simulink model "V2X_Core_SRI_coding_rate_symbol"  (R2023b)
settings: Solver=ode23tb  StartTime=0.0  StopTime=50  MaxStep=1e-2  RelTol=1e-3  AbsTol=1e-3
StopFcn:
  | run('saving.m')
values from neighbouring files (symbols this model uses):
  b = 1.6    [a2024_v2x_matlab_6veh.m]
  m = 2000    [a2024_v2x_matlab_6veh.m]
  mEgo = 1500    [a2024_v2x_matlab_6veh.m]
  Mode = 1    [a2024_v2x_matlab_6veh.m]    (also in v2x_matlab.m; v2x_matlabV2.m; v2x_matlab_6veh.m; v2x_matlab_R.m)
  RefSpeed = 90/3.6    (= 25)    [v2x_matlabV2.m]    (also in v2x_matlab_R.m)
  RelDistThreshold = 300    [v2x_matlabV2.m]    (also in v2x_matlab_R.m)
  s = RandStream("dsfmt19937","Seed",15)    [v2x_matlab.m]
  sampleTime = 0.1    [a2024_v2x_matlab_6veh.m]    (also in v2x_matlab.m; v2x_matlabV2.m; v2x_matlab_6veh.m; v2x_matlab_R.m)
  waypoints = [egoWP(:,2) egoWP(:,1), zeroforwp]    [a2024_v2x_matlab_6veh.m]    (also in misc.m = data.data.ActorSpecifications(1,1).Waypoints(:,[1,2]); v2x_matlab.m = data.data.ActorSpecifications(1,1).Waypoints(:,[1,2]); v2x_matlabV2.m = [5 -1.6 0; v2x_matlab_R.m = [5 -1.6 0)
  ZeroActors = struct(     'ActorID',0,     'Position', [1000 1000 1000],      'Velocity', [0 0 0],      'Roll', 0,      'Pitch', 0,      'Yaw', 0,      'AngularVelocity', [0 0 0])    [v2x_matlabV2.m]    (also in v2x_matlab_R.m)
undefined symbols (not defined in the file or in its folder): Battery, Brakes, Control, DiscIntNeverNeededParam, doppler, Drivetrain, ElectricMotor, Env, FB_flag, Init, SNR_value_list, Vehicle, Wheels
libraries: simulink x45, commofdm x29, commdigbbndam3 x15, commchan3 x14, simulink_extras x13, commcnvcod2 x12, commdigbbndpm3 x11, commblkintrlv2 x10, dspmathops x6, sharedtransform x6, autolibutils x6, autolibsharedcoupling x4
(part 4 of 8)

== system V2X_Core_SRI_coding_rate_symbol/DSRC/Subsystem7 ==
  VehicleID : Inport
  Trigger : Inport  Port=2
  Actors : Inport  Port=3
  Ego : Inport  Port=4
  Pilot1 : Inport  Port=5
  1/2 QPSK : Subsystem  Commented=on  TreatAsAtomicUnit=on
  64 QAM : Subsystem  Commented=on  TreatAsAtomicUnit=on
  Add : Sum  Commented=on  Inputs=+-
  Bus Creator : BusCreator  Inputs=2
  Bus Selector : BusSelector  Commented=on  OutputSignals=Actors
  Bus Selector1 : BusSelector  Commented=on  OutputSignals=Position,Velocity
  Constant : Constant  Commented=on  Value=0
  Integer to Bit Converter2 : simulink/Logic and Bit Operations/Integer to Bit Converter  Commented=on  nbits=16  signedInputValues=Signed  bitOrder=MSB first  outDtype=boolean
  MATLAB Function1 : MATLAB Function  Commented=on  TreatAsAtomicUnit=on
  MATLAB Function2 : MATLAB Function  Commented=on  TreatAsAtomicUnit=on
  MATLAB Function3 : MATLAB Function  Commented=on  TreatAsAtomicUnit=on  SystemSampleTime=0.01
  MIMO Fading Channel : commchan3/MIMO Fading Channel  Commented=on  InheritSampleRate=on  SampleRate=1  PathDelays=0  AveragePathGains=0  NormalizePathGains=on  FadingDistribution=Rayleigh  KFactor=3  DirectPathDopplerShift=0  DirectPathInitialPhase=0  MaximumDopplerShift=0.001  DopplerSpectrum=doppler('Jakes')  SpatialCorrelationSpecification=None  SpatialCorrelationMatrix=[1 0 0 0; 0 1 0 0; 0 0 1 0; 0 0 0 1]  NumTransmitAntennas=1  NumReceiveAntennas=1  TransmitCorrelationMatrix=[1 0; 0 1]  ReceiveCorrelationMatrix=[1 0; 0 1]  AntennaSelection=Off  NormalizeChannelOutputs=on  PathGainsOutputPort=off  SimulateUsing=Interpreted execution  FadingTechnique=Filtered Gaussian noise  NumSinusoids=48  InitialTimeSource=Property  InitialTime=0  RandomStream=mt19937ar with seed  Seed=73  Visualization=Off  AntennaPairsToDisplay=[ 1, 1 ]  PathsForDopplerDisplay=1  SamplesToDisplay=25%
  SISO Fading Channel : commchan3/SISO Fading Channel  Commented=on  InheritSampleRate=off  SampleRate=5.9e9  PathDelays=0  AveragePathGains=0  NormalizePathGains=on  FadingDistribution=Rayleigh  KFactor=3  DirectPathDopplerShift=0  DirectPathInitialPhase=0  MaximumDopplerShift=0.001  DopplerSpectrum=doppler('Jakes')  RandomStream=mt19937ar with seed  Seed=73  PathGainsOutputPort=off  ChannelFilterDelayOutputPort=off  SimulateUsing=Interpreted execution  Visualization=Off  PathsForDopplerDisplay=1  SamplesToDisplay=25%
  Scope : Scope  Commented=on
  Scope1 : Scope  Commented=on
  Selector : Selector  Commented=on  InputPortWidth=1  IndexOptions=Index vector (dialog)  Indices=1  OutputSizes=1
  Selector1 : Selector  Commented=on  InputPortWidth=3  IndexOptions=Index vector (dialog)  Indices=1  OutputSizes=1
  Selector2 : Selector  Commented=on  InputPortWidth=3  IndexOptions=Index vector (dialog)  Indices=1  OutputSizes=1
  Variant Sink : VariantSink  Commented=on
  Variant Source : VariantSource  Commented=on
  dB Conversion : dspmathops/dB Conversion  Commented=on  dBtype=dB  intype=Amplitude  R=1  fuzz=off
      settings: LibrarySourceBlock=commutil2/dB Conversion
  SentValues : Outport
  VehicleData : Outport  Port=2
  V1 : Outport  Port=3
  PosX : Outport  Port=4
  VelX : Outport  Port=5
  Actor5 : Outport  Port=6
  wires:
  MATLAB Function1/1(Actor) -> MATLAB Function3/1(input), Integer to Bit Converter2/1
  Ego/1 -> MATLAB Function1/3(EgoData)
  Actors/1 -> Bus Selector/1, MATLAB Function1/1(busActors3Test1)
  VehicleID/1 -> MATLAB Function1/2(VehicleID)
  MATLAB Function1/2(VehicleData) -> VehicleData/1
  MATLAB Function1/3(counter_out) -> V1/1
  Trigger/1 -> MATLAB Function1/Trigger
  MATLAB Function1/5(Pr) -> Bus Creator/2, Scope1/1  "ActorRxPower"
  MATLAB Function1/4(SNR) -> Add/1
  Add/1 -> MATLAB Function2/2(SNR), Scope/1
  Selector1/1 -> PosX/1
  Bus Selector/1 -> Selector/1  "<Actors>"
  Selector/1 -> Bus Selector1/1
  Bus Selector1/1 -> Selector1/1  "<Position>"
  Bus Selector1/2 -> Selector2/1  "<Velocity>"
  Selector2/1 -> VelX/1
  Variant Sink/2 -> 1/2 QPSK/1(Bits)
  Pilot1/1 -> 64 QAM/2(Pilot), 1/2 QPSK/2(Pilot)
  Integer to Bit Converter2/1 -> Variant Sink/1
  Variant Source/1 -> MATLAB Function2/1(modulated)
  1/2 QPSK/1(Modulated) -> Variant Source/2
  64 QAM/1(Modulated) -> Variant Source/1
  Variant Sink/1 -> 64 QAM/1(Bits)
  Constant/1 -> Add/2
  MATLAB Function2/1(signal) -> Bus Creator/1  "ActorData"
  Bus Creator/1 -> Actor5/1
  MATLAB Function3/1(Actors) -> SentValues/1

== system V2X_Core_SRI_coding_rate_symbol/DSRC/Subsystem8 ==
  VehicleID : Inport
  Trigger : Inport  Port=2
  Actors : Inport  Port=3
  Ego : Inport  Port=4
  Pilot1 : Inport  Port=5
  1/2 QPSK : Subsystem  Commented=on  TreatAsAtomicUnit=on
  64 QAM : Subsystem  Commented=on  TreatAsAtomicUnit=on
  Add : Sum  Commented=on  Inputs=+-
  Bus Creator : BusCreator  Inputs=2
  Bus Selector : BusSelector  Commented=on  OutputSignals=Actors
  Bus Selector1 : BusSelector  Commented=on  OutputSignals=Position,Velocity
  Constant : Constant  Commented=on  Value=0
  Integer to Bit Converter2 : simulink/Logic and Bit Operations/Integer to Bit Converter  Commented=on  nbits=16  signedInputValues=Signed  bitOrder=MSB first  outDtype=boolean
  MATLAB Function1 : MATLAB Function  Commented=on  TreatAsAtomicUnit=on
  MATLAB Function2 : MATLAB Function  Commented=on  TreatAsAtomicUnit=on
  MATLAB Function3 : MATLAB Function  Commented=on  TreatAsAtomicUnit=on  SystemSampleTime=0.01
  MIMO Fading Channel : commchan3/MIMO Fading Channel  Commented=on  InheritSampleRate=on  SampleRate=1  PathDelays=0  AveragePathGains=0  NormalizePathGains=on  FadingDistribution=Rayleigh  KFactor=3  DirectPathDopplerShift=0  DirectPathInitialPhase=0  MaximumDopplerShift=0.001  DopplerSpectrum=doppler('Jakes')  SpatialCorrelationSpecification=None  SpatialCorrelationMatrix=[1 0 0 0; 0 1 0 0; 0 0 1 0; 0 0 0 1]  NumTransmitAntennas=1  NumReceiveAntennas=1  TransmitCorrelationMatrix=[1 0; 0 1]  ReceiveCorrelationMatrix=[1 0; 0 1]  AntennaSelection=Off  NormalizeChannelOutputs=on  PathGainsOutputPort=off  SimulateUsing=Interpreted execution  FadingTechnique=Filtered Gaussian noise  NumSinusoids=48  InitialTimeSource=Property  InitialTime=0  RandomStream=mt19937ar with seed  Seed=73  Visualization=Off  AntennaPairsToDisplay=[ 1, 1 ]  PathsForDopplerDisplay=1  SamplesToDisplay=25%
  SISO Fading Channel : commchan3/SISO Fading Channel  Commented=on  InheritSampleRate=off  SampleRate=5.9e9  PathDelays=0  AveragePathGains=0  NormalizePathGains=on  FadingDistribution=Rayleigh  KFactor=3  DirectPathDopplerShift=0  DirectPathInitialPhase=0  MaximumDopplerShift=0.001  DopplerSpectrum=doppler('Jakes')  RandomStream=mt19937ar with seed  Seed=73  PathGainsOutputPort=off  ChannelFilterDelayOutputPort=off  SimulateUsing=Interpreted execution  Visualization=Off  PathsForDopplerDisplay=1  SamplesToDisplay=25%
  Scope : Scope  Commented=on
  Scope1 : Scope  Commented=on
  Selector : Selector  Commented=on  InputPortWidth=1  IndexOptions=Index vector (dialog)  Indices=1  OutputSizes=1
  Selector1 : Selector  Commented=on  InputPortWidth=3  IndexOptions=Index vector (dialog)  Indices=1  OutputSizes=1
  Selector2 : Selector  Commented=on  InputPortWidth=3  IndexOptions=Index vector (dialog)  Indices=1  OutputSizes=1
  Variant Sink : VariantSink  Commented=on
  Variant Source : VariantSource  Commented=on
  dB Conversion : dspmathops/dB Conversion  Commented=on  dBtype=dB  intype=Amplitude  R=1  fuzz=off
      settings: LibrarySourceBlock=commutil2/dB Conversion
  SentValues : Outport
  VehicleData : Outport  Port=2
  V1 : Outport  Port=3
  PosX : Outport  Port=4
  VelX : Outport  Port=5
  Actor6 : Outport  Port=6
  wires:
  MATLAB Function3/1(Actors) -> SentValues/1
  Bus Creator/1 -> Actor6/1
  MATLAB Function2/1(signal) -> Bus Creator/1  "ActorData"
  Constant/1 -> Add/2
  Variant Sink/1 -> 64 QAM/1(Bits)
  64 QAM/1(Modulated) -> Variant Source/1
  1/2 QPSK/1(Modulated) -> Variant Source/2
  Variant Source/1 -> MATLAB Function2/1(modulated)
  Integer to Bit Converter2/1 -> Variant Sink/1
  Pilot1/1 -> 1/2 QPSK/2(Pilot), 64 QAM/2(Pilot)
  Variant Sink/2 -> 1/2 QPSK/1(Bits)
  Selector2/1 -> VelX/1
  Bus Selector1/2 -> Selector2/1  "<Velocity>"
  Bus Selector1/1 -> Selector1/1  "<Position>"
  Selector/1 -> Bus Selector1/1
  Bus Selector/1 -> Selector/1  "<Actors>"
  Selector1/1 -> PosX/1
  Add/1 -> Scope/1, MATLAB Function2/2(SNR)
  MATLAB Function1/4(SNR) -> Add/1
  MATLAB Function1/5(Pr) -> Scope1/1, Bus Creator/2  "ActorRxPower"
  Trigger/1 -> MATLAB Function1/Trigger
  MATLAB Function1/3(counter_out) -> V1/1
  MATLAB Function1/2(VehicleData) -> VehicleData/1
  VehicleID/1 -> MATLAB Function1/2(VehicleID)
  Actors/1 -> MATLAB Function1/1(busActors3Test1), Bus Selector/1
  Ego/1 -> MATLAB Function1/3(EgoData)
  MATLAB Function1/1(Actor) -> Integer to Bit Converter2/1, MATLAB Function3/1(input)

== system V2X_Core_SRI_coding_rate_symbol/DelayMessage1/Subsystem ==
  Queue : Inport
  Trigger : TriggerPort  VariantControl=(inherit)  PortDimensions=1
  Receive : Receive  InputPortMessageModes=m  UseInternalQueue=off  QueueOverwriting=on  QueueLength=1  QueueType=LIFO
  Out : Outport
  wires:
  Queue/1 -> Receive/1
  Receive/1 -> Out/1

== system V2X_Core_SRI_coding_rate_symbol/VehicleDynamic/AccelerationToTrq ==
  IntendedLongAcc[m/s**2] : Inport
  LongVehSpd[m/s] : Inport  Port=2
  UnloadedTireRadius[m] : Inport  Port=3
  OverallMass[kg] : Inport  Port=4
  EngInrt[kg*m**2] : Inport  Port=5
  WheelRotAxisInrt[kg*m**2] : Inport  Port=6
  TireMaxRollResistanceTrq[Nm] : Inport  Port=7
  AeroFrc(VehSys)[N] : Inport  Port=8
  TorqueRatio[-] : Inport  Port=9
  ZeroAccPedalTrq[Nm] : Inport  Port=10
  FullAccPedalTrq[Nm] : Inport  Port=11
  StandstillSwitch[0;1] : Inport  Port=12
  MaxMainBrakePress[Pa] : Inport  Port=13
  BrakeTrqPressRatio[m**3] : Inport  Port=14
  CalculateIntendedTorque : Subsystem
  CalculateMainBrakePressure : Subsystem
  Scope : Scope
  TorqueSplitter : Subsystem
  IntendedDriveTrq[Nm] : Outport
  IntendedMainBrakePress[Pa] : Outport  Port=2
  IntendedTrq[Nm] : Outport  Port=3
  wires:
  EngInrt[kg*m**2]/1 -> CalculateIntendedTorque/4(EngInrt[kg*m**2])
  TorqueSplitter/2(IntendedBrakeTrq[Nm]) -> CalculateMainBrakePressure/1(IntendedBrakeTrq[Nm])
  OverallMass[kg]/1 -> CalculateIntendedTorque/3(OverallMass[kg])
  FullAccPedalTrq[Nm]/1 -> TorqueSplitter/4(FullAccPedalTrq[Nm])
  TorqueRatio[-]/1 -> TorqueSplitter/3(TorqueRatio[-]), CalculateIntendedTorque/8(TorqueRatio[-])
  StandstillSwitch[0;1]/1 -> CalculateMainBrakePressure/2(StandstillSwitch[0;1])
  TireMaxRollResistanceTrq[Nm]/1 -> CalculateIntendedTorque/6(TireMaxRollResistanceTrq[Nm])
  IntendedLongAcc[m/s**2]/1 -> CalculateIntendedTorque/1(IntendedLongAcc[m/s**2])
  ZeroAccPedalTrq[Nm]/1 -> TorqueSplitter/2(ZeroAccPedalTrq[Nm]), CalculateIntendedTorque/9(MinEngTrq[Nm])
  UnloadedTireRadius[m]/1 -> CalculateIntendedTorque/2(UnloadedTireRadius[m])
  TorqueSplitter/1(IntendedDriveTrq[Nm]) -> IntendedDriveTrq[Nm]/1
  LongVehSpd[m/s]/1 -> CalculateMainBrakePressure/3(LongVehSpd[m/s])
  BrakeTrqPressRatio[m**3]/1 -> CalculateMainBrakePressure/5(BrakeTrqPressRatio[m**3])
  WheelRotAxisInrt[kg*m**2]/1 -> CalculateIntendedTorque/5(WheelRotAxisInrt[kg*m**2])
  MaxMainBrakePress[Pa]/1 -> CalculateMainBrakePressure/4(MaxMainBrakePress[Pa])
  AeroFrc(VehSys)[N]/1 -> CalculateIntendedTorque/7(AeroFrc(VehSys)[N])
  CalculateMainBrakePressure/1(IntendedMainBrakePress[Pa]) -> Scope/1, IntendedMainBrakePress[Pa]/1
  CalculateIntendedTorque/1(IntendedTrq[Nm]) -> IntendedTrq[Nm]/1, TorqueSplitter/1("IntendedTrq[Nm] ")

== system V2X_Core_SRI_coding_rate_symbol/VehicleDynamic/DrivetrainControlUnit ==
  note: Copyright 2015-2022 The MathWorks, Inc.
  AccelPdl : Inport  OutDataTypeStr=double  PortDimensions=1
  BcuBrkPrsCmd : Inport  Port=2  OutDataTypeStr=double  PortDimensions=4
  VehSpdFdbk : Inport  Port=3  OutDataTypeStr=double  PortDimensions=1
  EMSpd : Inport  Port=4  OutDataTypeStr=double  PortDimensions=1
  BMSSOC : Inport  Port=5
  BattPackVolt : Inport  Port=6
  BMSDischrgCurrLmt : Inport  Port=7
  BMSChrgCurrLmt : Inport  Port=8
  IntendedDriveTrq[Nm] : Inport  Port=9
  Accel Pedal to Traction Wheel Torque Request : Subsystem  InitFcn=[~]=autosharedicon('autolibinternalvvblock',gcb,0,'6');
  Brake Pedal to Total Braking Pressure Request : Subsystem
  Constant : Constant  Value=0
  Motor Torque Arbitration and Power Management : Subsystem
  Power Limit Calculations : Subsystem
  Series Regen Braking : Subsystem
  Subsystem2 : Subsystem
  Terminator : Terminator
  EMTrqCmd : Outport  OutDataTypeStr=double  PortDimensions=1  VectorParamsAs1DForOutWhenUnconnected=off
  DcuBrkPrsCmd : Outport  Port=2  OutDataTypeStr=double  PortDimensions=4  VectorParamsAs1DForOutWhenUnconnected=off
  wires:
  BMSSOC/1 -> Subsystem2/1(SOC)
  [EMSpd] -> Motor Torque Arbitration and Power Management/5(EMSpd)
  BMSDischrgCurrLmt/1 -> Power Limit Calculations/2(BMSDischrgCurrLmt)
  Series Regen Braking/1(" EMTrqCmdRegen") -> Motor Torque Arbitration and Power Management/7(EMTrqCmdRegen)  "EMTrqCmdRegen"
  Brake Pedal to Total Braking Pressure Request/1(BrkPrsReq) -> Series Regen Braking/4("BrkPrsReq ")
  AccelPdl/1 -> [AccelPdl], Accel Pedal to Traction Wheel Torque Request/1(AccelPdl)
  Constant/1 -> Brake Pedal to Total Braking Pressure Request/2(Park)
  BMSChrgCurrLmt/1 -> Power Limit Calculations/3(BMSChrgCurrLmt)
  BcuBrkPrsCmd/1 -> Brake Pedal to Total Braking Pressure Request/1(BcuBrkPrsCmd)  "DecelPdl"
  BattPackVolt/1 -> Power Limit Calculations/1(PackVolt)
  VehSpdFdbk/1 -> Series Regen Braking/2(VehSpd)  "VehSpd"
  EMSpd/1 -> Series Regen Braking/3("EMSpd "), [EMSpd]  "EMSpd"
  [EMSpd] -> Accel Pedal to Traction Wheel Torque Request/2(EMSpd)
  Power Limit Calculations/2(BattPwrChrgLmt) -> Motor Torque Arbitration and Power Management/4("BattPwrChrgLmt ")  "BattPwrChrgLmt"
  Power Limit Calculations/1(BattPwrDischrgLmt) -> Motor Torque Arbitration and Power Management/3(BattPwrDisChrgLmt)  "BattPwrDischrgLmt"
  [AccelPdl] -> Motor Torque Arbitration and Power Management/2(AccelPdl)
  Motor Torque Arbitration and Power Management/1(EMTrqCmdFinal) -> EMTrqCmd/1  "EMTrqCmd"
  Subsystem2/1(BattSOC) -> Series Regen Braking/1(BattSoc), Motor Torque Arbitration and Power Management/6(SOC)  "SOC"
  IntendedDriveTrq[Nm]/1 -> Motor Torque Arbitration and Power Management/1(EMTrqCmdTrac)
  Accel Pedal to Traction Wheel Torque Request/1(TrqCmd) -> Terminator/1
  Series Regen Braking/2(" BrkCmd") -> DcuBrkPrsCmd/1  "BrkCmd"

== system V2X_Core_SRI_coding_rate_symbol/VehicleDynamic/Enabled Subsystem ==
  In1 : Inport
  Enable : EnablePort
  Out1 : Outport
  wires:
  In1/1 -> Out1/1

== system V2X_Core_SRI_coding_rate_symbol/VehicleDynamic/FiveSteteABS-TCS ==
  note: Copyright 2022 The MathWorks, Inc.
  AccelFdbk : Inport  OutDataTypeStr=double  PortDimensions=1
  DecelFdbk : Inport  Port=2  OutDataTypeStr=double  PortDimensions=1
  Acc : Inport  Port=3  OutDataTypeStr=double
  Omega : Inport  Port=4  OutDataTypeStr=double  PortDimensions=4
  BrkPrs : Inport  Port=5  OutDataTypeStr=double  PortDimensions=4
  ABSCtrlForEach : Subsystem  mask(Five-State ABS Control){Re=Wheels.EffectiveRadius, KappaOpt=-0.12, WhlAccelOpt=[-9.8,-9.8,-20,-20], v1=0, v5=0.55, v4=1, a2=-1.5, b=-1.5, A=4.5, a1=3.6, aMode=2}
      mask prompts: Re "Wheel effective radius, Re [m]:"; KappaOpt "Desired wheel slip ratio, KappaOpt [-]:"; WhlAccelOpt "Desired wheel acceleration, WhlAccelOpt [m/s^2]:"; v1 "Braking realease command, v1 [-]:"; v5 "Braking hold command, v5 [-]:"; v4 "Braking add command, v4 [-]:"; a2 "Threshold of State 1, a2 [m/s^2]:"; b "Threshold of State 2, b [m/s^2]:"; A "Threshold of State 3 and 4, A [m/s^2]:"; a1 "Threshold of State 5, a1 [m/s^2]:"
      mask help: This block determines brake pressure varying rate for each wheel once the ABS controller is activated. During ABS control, only wheel speed is directly regulated.
      mask init:
      | [~]=vehdynicon('vehdynblk',gcb);
      mask DialogControl vehParamGroup Prompt: Vehicle Parameter
      mask DialogControl ParameterGroupVar Prompt: Desired Control Parameters
      mask DialogControl Container3 Prompt: Braking Pressure Rates
      mask DialogControl Container4 Prompt: Wheel Acceleration Thresholds
  Data Type Conversion : DataTypeConversion  OutDataTypeStr=boolean  SaturateOnIntegerOverflow=off  RndMeth=Floor
  Logical Operator : Logic  Operator=OR  AllPortsSameDT=off  OutDataTypeStr=boolean
  Sum : Sum  Inputs=|++
  Switch : Switch  Criteria=u2 > Threshold  SaturateOnIntegerOverflow=off  InputSameDT=off
  TCSCtrlForEach : Subsystem  mask(Five-State TCS Control){Re=Wheels.EffectiveRadius, KappaOpt=0.12, WhlAccelOpt=[11, 11, 11, 11], v1=1.5, v5=-0.5, v4=-1.2, a2=-6, b=-10, A=-11, a1=-9, aMode=2}
      mask prompts: Re "Wheel effective radius, Re [m]:"; KappaOpt "Desired wheel slip ratio, KappaOpt [-]:"; WhlAccelOpt "Desired wheel acceleration, WhlAccelOpt [m/s^2]:"; v1 "Braking pressure rising rate, v1 [-]:"; v5 "Secondary braking pressure declining rate, v5 [-]:"; v4 "Braking pressure declining rate, v4 [-]:"; a2 "Threshold of State 1, a2 [m/s^2]:"; b "Threshold of State 2, b [m/s^2]:"; A "Threshold of State 3 and 4, A [m/s^2]:"; a1 "Threshold of State 5, a1 [m/s^2]:"
      mask help: This block determines brake pressure varying rate for each wheel once the TCS controller is activated. During TCS control, only wheel speed is directly regulated.
      mask init:
      | [~]=vehdynicon('vehdynblk',gcb);
      mask DialogControl vehParamGroup Prompt: Vehicle Parameter
      mask DialogControl ParameterGroupVar Prompt: Desired Control Parameters
      mask DialogControl Container3 Prompt: Braking Pressure Rates
      mask DialogControl Container4 Prompt: Wheel Acceleration Thresholds
  Wheel Accel and Slip Estimator1 : Subsystem
  BrkPrsCmd : Outport  OutDataTypeStr=double  PortDimensions=4
  ABSFlag : Outport  Port=2  OutDataTypeStr=boolean  PortDimensions=4
  TCSFlag : Outport  Port=3  OutDataTypeStr=double  PortDimensions=4
  wires:
  Sum/1 -> Switch/1
  Wheel Accel and Slip Estimator1/2(<Kappa>) -> TCSCtrlForEach/2(WhlSlip), ABSCtrlForEach/3(WhlSlip)
  Wheel Accel and Slip Estimator1/1(<WhlAccel>) -> TCSCtrlForEach/1(WhlAccel), ABSCtrlForEach/2(WhlAccel)
  AccelFdbk/1 -> TCSCtrlForEach/3(AccelFdbk)
  Acc/1 -> Wheel Accel and Slip Estimator1/2(Accel)
  BrkPrs/1 -> TCSCtrlForEach/4(PbFdbk)
  TCSCtrlForEach/2(BrkFlag) -> TCSFlag/1, Logical Operator/2
  ABSCtrlForEach/1(BrkCtrl) -> Sum/1
  ABSCtrlForEach/2(BrkFlag) -> Data Type Conversion/1, Logical Operator/1
  Switch/1 -> BrkPrsCmd/1
  Data Type Conversion/1 -> ABSFlag/1
  Logical Operator/1 -> Switch/2
  Omega/1 -> Wheel Accel and Slip Estimator1/1(Omega)
  TCSCtrlForEach/1(BrkCtrl) -> Sum/2
  Wheel Accel and Slip Estimator1/3(<xdot>) -> ABSCtrlForEach/4(VehSpd)
  DecelFdbk/1 -> Switch/3, ABSCtrlForEach/1(Pref)

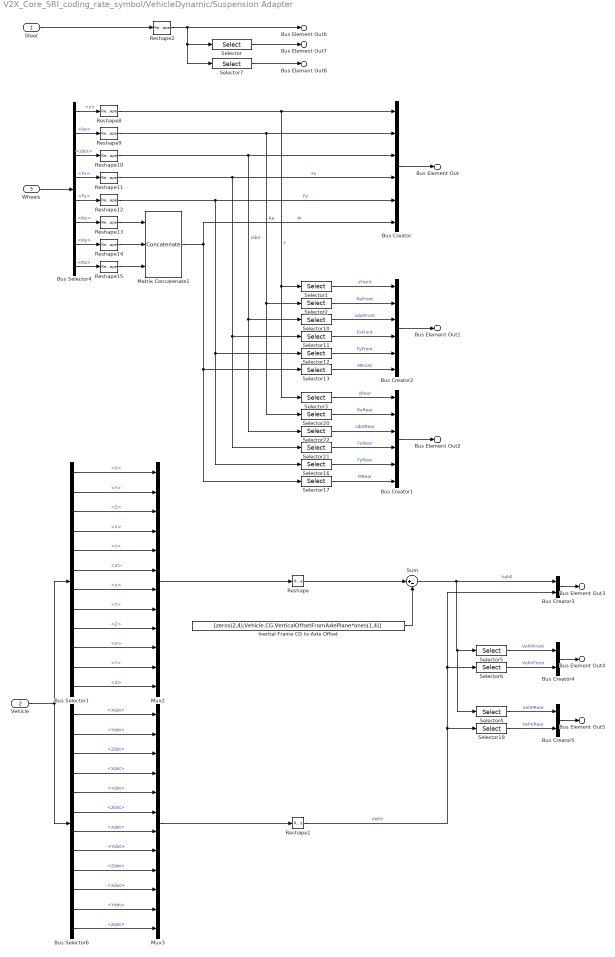
== system V2X_Core_SRI_coding_rate_symbol/VehicleDynamic/Suspension Adapter ==
  Steer : Inport
  Vehicle : Inport  Port=2
  Wheels : Inport  Port=3
  Bus Creator : BusCreator  Inputs=6
  Bus Creator1 : BusCreator  Inputs=6
  Bus Creator2 : BusCreator  Inputs=6
  Bus Creator3 : BusCreator  Inputs=2
  Bus Creator4 : BusCreator  Inputs=2
  Bus Creator5 : BusCreator  Inputs=2
  Bus Selector1 : BusSelector  OutputSignals=InertFrm.FrntAxl.Lft.Disp.X,InertFrm.FrntAxl.Lft.Disp.Y,InertFrm.FrntAxl.Lft.Disp.Z,InertFrm.FrntAxl.Rght.Disp.X,InertFrm.FrntAxl.Rght.Disp.Y,InertFrm.FrntAxl.Rght.Disp.Z,InertFrm.RearAxl.Lft.Disp.X,InertFrm.RearAxl.Lft.Disp.Y,InertFrm.RearAxl.Lft.Disp.Z,InertFrm.RearAxl.Rght.Disp.X,InertFrm.RearAxl.Rght.Disp.Y,InertFrm.RearAxl.Rght.Disp.Z
  Bus Selector4 : BusSelector  OutputSignals=SuspFrame.z,SuspFrame.Re,SuspFrame.zdot,SuspFrame.Fx,SuspFrame.Fy,SuspFrame.Mx,SuspFrame.My,SuspFrame.Mz
  Bus Selector6 : BusSelector  OutputSignals=InertFrm.FrntAxl.Lft.Vel.Xdot,InertFrm.FrntAxl.Lft.Vel.Ydot,InertFrm.FrntAxl.Lft.Vel.Zdot,InertFrm.FrntAxl.Rght.Vel.Xdot,InertFrm.FrntAxl.Rght.Vel.Ydot,InertFrm.FrntAxl.Rght.Vel.Zdot,InertFrm.RearAxl.Lft.Vel.Xdot,InertFrm.RearAxl.Lft.Vel.Ydot,InertFrm.RearAxl.Lft.Vel.Zdot,InertFrm.RearAxl.Rght.Vel.Xdot,InertFrm.RearAxl.Rght.Vel.Ydot,InertFrm.RearAxl.Rght.Vel.Zdot
  Inertial Frame CG to Axle Offset : Constant  Value=[zeros(2,4);Vehicle.CG.VerticalOffsetFromAxlePlane*ones(1,4)]
  Matrix Concatenate1 : Concatenate  NumInputs=3  Mode=Multidimensional array
  Mux2 : Mux  Inputs=12
  Mux3 : Mux  Inputs=12
  Reshape : Reshape  OutputDimensionality=Customize  OutputDimensions=[3,4]
  Reshape1 : Reshape  OutputDimensionality=Customize  OutputDimensions=[3,4]
  Reshape{2,8..15} (9 alike) : Reshape  OutputDimensionality=Row vector (2-D)
  Selector{,1..2,10..12} (6 alike) : Selector  IndexOptions=Index vector (dialog)  Indices=[1 2]  OutputSizes=1
  Selector13 : Selector  NumberOfDimensions=2  IndexOptions=Select all,Index vector (dialog)  Indices=[1 2],[1 2]  OutputSizes=1,1
  Selector{3,7,16,20..22} (6 alike) : Selector  IndexOptions=Index vector (dialog)  Indices=[3 4]  OutputSizes=1
  Selector17 : Selector  NumberOfDimensions=2  IndexOptions=Select all,Index vector (dialog)  Indices=[1 2],[3 4]  OutputSizes=1,1
  Selector18 : Selector  NumberOfDimensions=2  IndexOptions=Select all,Index vector (dialog)  Indices=[1 2],[3 4]  OutputSizes=1,1
  Selector4 : Selector  NumberOfDimensions=2  IndexOptions=Select all,Index vector (dialog)  Indices=[1 2],[3 4]  OutputSizes=1,1
  Selector5 : Selector  NumberOfDimensions=2  IndexOptions=Select all,Index vector (dialog)  Indices=[1 2],[1 2]  OutputSizes=1,1
  Selector6 : Selector  NumberOfDimensions=2  IndexOptions=Select all,Index vector (dialog)  Indices=[1 2],[1 2]  OutputSizes=1,1
  Sum : Sum  Inputs=|+-
  Bus Element Out : Outport  PortName=WheelsSusp  Element=All
  Bus Element Out1 : Outport  PortName=WheelsSusp  Element=Front
  Bus Element Out2 : Outport  PortName=WheelsSusp  Element=Rear
  Bus Element Out3 : Outport  Port=2  PortName=VehSusp  Element=All
  Bus Element Out4 : Outport  Port=2  PortName=VehSusp  Element=Front
  Bus Element Out5 : Outport  Port=2  PortName=VehSusp  Element=Rear
  Bus Element Out6 : Outport  Port=3  PortName=SteeringAngles  Element=StrgAngAll
  Bus Element Out7 : Outport  Port=3  PortName=SteeringAngles  Element=StrgAngFront
  Bus Element Out8 : Outport  Port=3  PortName=SteeringAngles  Element=StrgAngRear
  wires:
  Reshape9/1 -> Selector2/1, Selector20/1, Bus Creator/2  "Re"
  Selector2/1 -> Bus Creator2/2  "ReFront"
  Selector13/1 -> Bus Creator2/6  "MFront"
  Selector11/1 -> Bus Creator2/4  "FxFront"
  Reshape12/1 -> Bus Creator/5, Selector12/1, Selector16/1  "Fy"
  Selector1/1 -> Bus Creator2/1  "zFront"
  Bus Creator/1 -> Bus Element Out/1
  Reshape11/1 -> Bus Creator/4, Selector11/1, Selector21/1  "Fx"
  Bus Creator1/1 -> Bus Element Out2/1
  Selector3/1 -> Bus Creator1/1  "zRear"
  Wheels/1 -> Bus Selector4/1
  Selector12/1 -> Bus Creator2/5  "FyFront"
  Matrix Concatenate1/1 -> Bus Creator/6, Selector13/1, Selector17/1  "M"
  Bus Selector4/5 -> Reshape12/1  "<Fy>"
  Bus Selector4/2 -> Reshape9/1  "<Re>"
  Reshape13/1 -> Matrix Concatenate1/1
  Reshape14/1 -> Matrix Concatenate1/2
  Bus Selector4/1 -> Reshape8/1  "<z>"
  Bus Creator2/1 -> Bus Element Out1/1
  Selector17/1 -> Bus Creator1/6  "MRear"
  Reshape15/1 -> Matrix Concatenate1/3
  Bus Selector4/7 -> Reshape14/1  "<My>"
  Bus Selector4/8 -> Reshape15/1  "<Mz>"
  Bus Selector4/4 -> Reshape11/1  "<Fx>"
  Bus Selector4/3 -> Reshape10/1  "<zdot>"
  Selector10/1 -> Bus Creator2/3  "zdotFront"
  Selector22/1 -> Bus Creator1/3  "zdotRear"
  Reshape10/1 -> Bus Creator/3, Selector10/1, Selector22/1  "zdot"
  Reshape8/1 -> Bus Creator/1, Selector1/1, Selector3/1  "z"
  Selector16/1 -> Bus Creator1/5  "FyRear"
  Selector21/1 -> Bus Creator1/4  "FxRear"
  Bus Selector4/6 -> Reshape13/1  "<Mx>"
  Selector20/1 -> Bus Creator1/2  "ReRear"
  Selector4/1 -> Bus Creator5/1  "VehPRear"
  Bus Creator4/1 -> Bus Element Out4/1
  Bus Selector6/1 -> Mux3/1  "<Xdot>"
  Bus Selector6/9 -> Mux3/9  "<Zdot>"
  Bus Selector1/10 -> Mux2/10  "<X>"
  Bus Selector1/8 -> Mux2/8  "<Y>"
  Reshape1/1 -> Bus Creator3/2, Selector6/1, Selector18/1  "VehV"
  Reshape/1 -> Sum/1
  Mux3/1 -> Reshape1/1
  Bus Selector1/5 -> Mux2/5  "<Y>"
  Bus Selector6/2 -> Mux3/2  "<Ydot>"
  Bus Selector1/2 -> Mux2/2  "<Y>"
  Bus Selector1/4 -> Mux2/4  "<X>"
  Bus Creator5/1 -> Bus Element Out5/1
  Bus Selector1/3 -> Mux2/3  "<Z>"
  Bus Selector1/9 -> Mux2/9  "<Z>"
  Bus Selector1/11 -> Mux2/11  "<Y>"
  Bus Selector6/11 -> Mux3/11  "<Ydot>"
  Bus Selector1/6 -> Mux2/6  "<Z>"
  Bus Selector6/8 -> Mux3/8  "<Ydot>"
  Inertial Frame CG to Axle Offset/1 -> Sum/2
  Bus Selector6/5 -> Mux3/5  "<Ydot>"
  Vehicle/1 -> Bus Selector6/1, Bus Selector1/1
  Bus Selector6/6 -> Mux3/6  "<Zdot>"
  Bus Selector6/10 -> Mux3/10  "<Xdot>"
  Selector18/1 -> Bus Creator5/2  "VehVRear"
  Selector6/1 -> Bus Creator4/2  "VehVFront"
  Bus Selector1/1 -> Mux2/1  "<X>"
  Bus Selector1/12 -> Mux2/12  "<Z>"
  Bus Creator3/1 -> Bus Element Out3/1
  Bus Selector1/7 -> Mux2/7  "<X>"
  Bus Selector6/4 -> Mux3/4  "<Xdot>"
  Selector5/1 -> Bus Creator4/1  "VehPFront"
  Bus Selector6/12 -> Mux3/12  "<Zdot>"
  Bus Selector6/3 -> Mux3/3  "<Zdot>"
  Bus Selector6/7 -> Mux3/7  "<Xdot>"
  Mux2/1 -> Reshape/1
  Sum/1 -> Selector4/1, Selector5/1, Bus Creator3/1  "VehP"
  Steer/1 -> Reshape2/1
  Reshape2/1 -> Selector7/1, Selector/1, Bus Element Out6/1
  Selector7/1 -> Bus Element Out8/1
  Selector/1 -> Bus Element Out7/1

== system V2X_Core_SRI_coding_rate_symbol/VehicleDynamic/Suspension Bus Creator ==
  Vehicle : Inport
  SuspensionInfo : Inport  Port=2
  Wheels : Inport  Port=3
  Add : Sum
  Bus Creator1 : BusCreator  Inputs=6
  Bus Creator2 : BusCreator  Inputs=2
  Bus Creator3 : BusCreator  Inputs=2
  Bus Selector1 : BusSelector  OutputSignals=BdyFrm.Cg.AngVel.r
  Bus Selector2 : BusSelector  OutputSignals=SuspFrame.z
  Bus Selector5 : BusSelector  OutputSignals=Front.VehF,Rear.VehF,Front.VehM,Rear.VehM,Front.WhlF,Rear.WhlF,Front.WhlAng,Rear.WhlAng
  Bus Selector6 : BusSelector  OutputSignals=BdyFrm.FrntAxl.Lft.Vel.xdot,BdyFrm.FrntAxl.Rght.Vel.xdot,BdyFrm.RearAxl.Lft.Vel.xdot,BdyFrm.RearAxl.Rght.Vel.xdot
  Bus Selector8 : BusSelector  OutputSignals=BdyFrm.FrntAxl.Lft.Vel.ydot,BdyFrm.FrntAxl.Rght.Vel.ydot,BdyFrm.RearAxl.Lft.Vel.ydot,BdyFrm.RearAxl.Rght.Vel.ydot
  Constant : Constant  Value=zeros(1,4)
  Matrix Concatenate{1,8..10} (4 alike) : Concatenate  Mode=Multidimensional array  ConcatenateDimension=2
  Matrix Concatenate3 : Concatenate  NumInputs=3  Mode=Multidimensional array
  Matrix Concatenate7 : Concatenate  NumInputs=3  Mode=Multidimensional array
  Mux : Mux
  Mux1 : Mux
  Reshape{,1..4} (5 alike) : Reshape  OutputDimensionality=Row vector (2-D)
  Selector24 : Selector  InputPortWidth=1  IndexOptions=Index vector (dialog)  Indices=[1 1 1 1]  OutputSizes=1
  SteerRates : Constant  Value=zeros(1,4)
  Suspension : Outport
  wires:
  Matrix Concatenate10/1 -> Bus Creator1/2  "Ang"
  Selector24/1 -> Reshape4/1
  Reshape3/1 -> Matrix Concatenate3/1, Matrix Concatenate3/2
  Add/1 -> Bus Creator1/6  "AngVel"
  Vehicle/1 -> Bus Selector1/1, Bus Selector8/1, Bus Selector6/1
  Mux1/1 -> Reshape1/1
  SteerRates/1 -> Reshape2/1
  Matrix Concatenate1/1 -> Bus Creator2/1  "F"
  Reshape1/1 -> Bus Creator1/5  "ydot"
  Bus Selector5/4 -> Matrix Concatenate8/2  "<VehM>"
  Matrix Concatenate3/1 -> Add/2
  Bus Creator1/1 -> Bus Creator3/2  "Whl"
  Bus Selector5/3 -> Matrix Concatenate8/1  "<VehM>"
  Matrix Concatenate8/1 -> Bus Creator2/2  "M"
  Bus Selector5/1 -> Matrix Concatenate1/1  "<VehF>"
  Matrix Concatenate7/1 -> Add/1
  SuspensionInfo/1 -> Bus Selector5/1
  Bus Creator2/1 -> Bus Creator3/1  "Veh"
  Bus Selector2/1 -> Bus Creator1/3  "<z>"
  Mux/1 -> Reshape/1
  Bus Selector5/5 -> Matrix Concatenate9/1  "<WhlF>"
  Bus Selector1/1 -> Selector24/1  "<r>"
  Constant/1 -> Reshape3/1
  Matrix Concatenate9/1 -> Bus Creator1/1  "F"
  Bus Selector5/6 -> Matrix Concatenate9/2  "<WhlF>"
  Reshape4/1 -> Matrix Concatenate3/3
  Reshape/1 -> Bus Creator1/4  "xdot"
  Reshape2/1 -> Matrix Concatenate7/3, Matrix Concatenate7/2, Matrix Concatenate7/1
  Bus Selector5/7 -> Matrix Concatenate10/1  "<WhlAng>"
  Bus Selector5/2 -> Matrix Concatenate1/2  "<VehF>"
  Bus Selector5/8 -> Matrix Concatenate10/2  "<WhlAng>"
  Wheels/1 -> Bus Selector2/1
  Bus Creator3/1 -> Suspension/1
  Bus Selector6/1 -> Mux/1  "<xdot>"
  Bus Selector6/2 -> Mux/2  "<xdot>"
  Bus Selector6/3 -> Mux/3  "<xdot>"
  Bus Selector6/4 -> Mux/4  "<xdot>"
  Bus Selector8/1 -> Mux1/1  "<ydot>"
  Bus Selector8/2 -> Mux1/2  "<ydot>"
  Bus Selector8/3 -> Mux1/3  "<ydot>"
  Bus Selector8/4 -> Mux1/4  "<ydot>"

== system V2X_Core_SRI_coding_rate_symbol/VehicleDynamic/Suspension to Chasiss Transforms ==
  Suspension : Inport
  VehFdbk : Inport  Port=2
  Add : Sum  Inputs=+-
  Add1 : Sum
  Bus Selector1 : BusSelector  OutputSignals=BdyFrm.Cg.DCM
  Bus Selector2 : BusSelector  OutputSignals=BdyFrm.Cg.Acc.xddot,BdyFrm.Cg.Vel.ydot,BdyFrm.Cg.AngVel.r,BdyFrm.Cg.Acc.yddot,BdyFrm.Cg.Vel.xdot,BdyFrm.Cg.AngVel.r
  Bus Selector3 : BusSelector  OutputSignals=Whl.z,Veh.F,Veh.M
  Bus Selector4 : BusSelector  OutputSignals=InertFrm.Cg.Ang.phi,InertFrm.Cg.Ang.theta,InertFrm.Cg.Ang.psi  OutputAsBus=on
  Bus Selector6 : BusSelector  OutputSignals=InertFrm.Geom.Disp.X,InertFrm.Geom.Disp.Y,InertFrm.Geom.Disp.Z  OutputAsBus=on
  Bus to Vector3 : BusToVector
  Bus to Vector5 : BusToVector
  Bushings : autolibutils/Cont LPF  wc=40*pi  AbsoluteTolerance=auto  aMode=2
  Estimated Unsprung Mass Orientation : MATLAB Function  TreatAsAtomicUnit=on  mask{trackW=Vehicle.TrackWidthFront, wheelB=Vehicle.CG.LongDistFrontAxle +  Vehicle.CG.LongDistRearAxle}
      mask prompts: trackW "Vehicle track width, trackW [m]:"; wheelB "Vehicle wheelbase, wheelB [m]:"
      mask help: This block converts wheel ground height information into estimates of vehicle pitch, roll angles and vertical height in order to help in the visualization 3DOF based simulations with changes in terrain. Note that the resulting signals are only used as a visualization aid and do not account for the physical affects of the vehicle interacting with variable terrain or changes in orientation.
  Product : Product
  Product1 : Product
  Susp2Body : Subsystem
  Terminator6 : Terminator
  Unary Minus : UnaryMinus
  Unsprung Masses : Gain  Gain=sum([Vehicle.UnsprungMassFrontAxle/2 Vehicle.UnsprungMassFrontAxle/2 Vehicle.UnsprungMassRearAxle/2 Vehicle.UnsprungMassRearAxle/2])  Multiplication=Matrix(u*K)
  Vector Concatenate : Concatenate
  Vector Concatenate1 : Concatenate
  Vertical : Constant  Value=0
  FsB : Outport
  MsB : Outport  Port=2
  Fext : Outport  Port=3
  wires:
  Bus Selector6/1 -> Bus to Vector5/1
  Bus Selector3/2 -> Susp2Body/4(Fs)  "<F>"
  VehFdbk/1 -> Bus Selector2/1, Bus Selector1/1, Bus Selector6/1, Bus Selector4/1
  Bus Selector3/3 -> Susp2Body/5(Ms)  "<M>"
  Bus to Vector3/1 -> Estimated Unsprung Mass Orientation/1(angleIn), Susp2Body/2(VehAng)
  Bus Selector1/1 -> Susp2Body/1(DCM)  "<DCM>"
  Bus to Vector5/1 -> Estimated Unsprung Mass Orientation/2(GemoXYZIn)
  Suspension/1 -> Bus Selector3/1
  Bus Selector4/1 -> Bus to Vector3/1
  Estimated Unsprung Mass Orientation/2(GeomXYZ) -> Terminator6/1
  Bus Selector3/1 -> Estimated Unsprung Mass Orientation/3(Ground)  "<z>"
  Estimated Unsprung Mass Orientation/1(angles) -> Susp2Body/3(SuspAng)
  Susp2Body/2(MsB) -> MsB/1
  Bushings/1 -> Unsprung Masses/1
  Vector Concatenate1/1 -> Bushings/1
  Unsprung Masses/1 -> Vector Concatenate/1
  Susp2Body/1(FsB) -> FsB/1
  Vector Concatenate/1 -> Unary Minus/1
  Vertical/1 -> Vector Concatenate/2
  Bus Selector2/2 -> Product/1  "<ydot>"
  Bus Selector2/3 -> Product/2  "<r>"
  Bus Selector2/5 -> Product1/1  "<xdot>"
  Bus Selector2/6 -> Product1/2  "<r>"
  Add/1 -> Vector Concatenate1/1
  Product/1 -> Add/2
  Product1/1 -> Add1/2
  Bus Selector2/4 -> Add1/1  "<yddot>"
  Add1/1 -> Vector Concatenate1/2
  Bus Selector2/1 -> Add/1  "<xddot>"
  Unary Minus/1 -> Fext/1

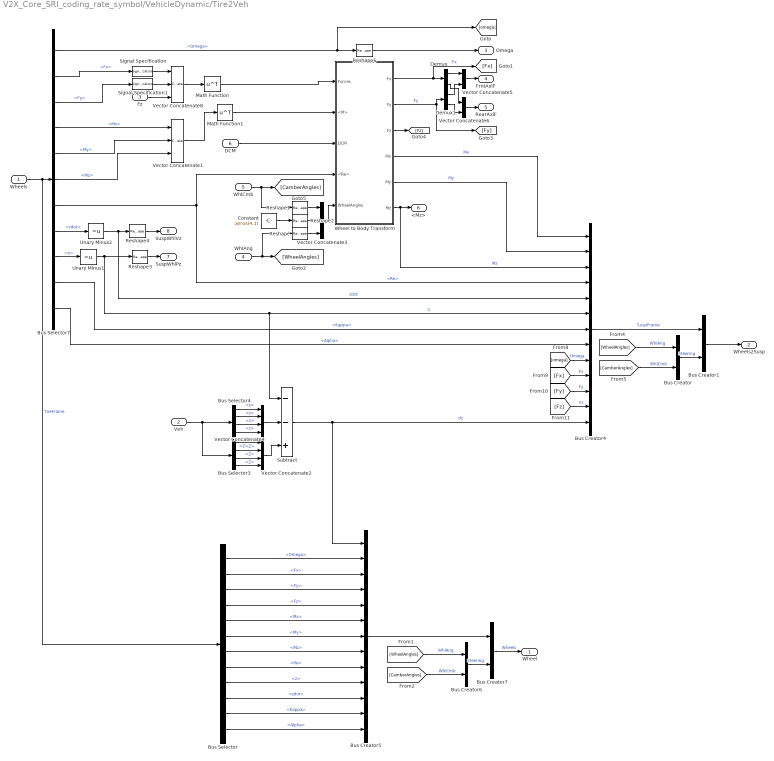
== system V2X_Core_SRI_coding_rate_symbol/VehicleDynamic/Tire2Veh ==
  Wheels : Inport
  Veh : Inport  Port=2
  Fz : Inport  Port=3  PortDimensions=4
  WhlAng : Inport  Port=4
  WhlCmb : Inport  Port=5
  DCM : Inport  Port=6
  Bus Creator{,1,6..7} (4 alike) : BusCreator  Inputs=2
  Bus Creator4 : BusCreator  Inputs=13
  Bus Creator5 : BusCreator  Inputs=13
  Bus Selector : BusSelector  OutputSignals=Omega,Fx,Fy,Fz,Mx,My,Mz,Re,z,zdot,Kappa,Alpha
  Bus Selector3 : BusSelector  OutputSignals=InertFrm.FrntAxl.Lft.Disp.Z,InertFrm.FrntAxl.Rght.Disp.Z,InertFrm.RearAxl.Lft.Disp.Z,InertFrm.RearAxl.Rght.Disp.Z
  Bus Selector4 : BusSelector  OutputSignals=BdyFrm.FrntAxl.Lft.Disp.z,BdyFrm.FrntAxl.Rght.Disp.z,BdyFrm.RearAxl.Lft.Disp.z,BdyFrm.RearAxl.Rght.Disp.z
  Bus Selector7 : BusSelector  OutputSignals=Omega,Fx,Fy,Mx,My,Mz,Re,zdot,z,Kappa,Alpha
  Constant : Constant  Value=zeros(4,1)
  Demux : Demux  Outputs=[2,2]
  Demux1 : Demux  Outputs=[2,2]
  Math Function : Math  Operator=transpose  SignedPower=on
  Math Function1 : Math  Operator=transpose  SignedPower=on
  Reshape{,1..4} (5 alike) : Reshape  OutputDimensionality=Row vector (2-D)
  Reshape6 : Reshape  OutputDimensionality=Customize  OutputDimensions=[2,2]
  Signal Specification : SignalSpecification  Dimensions=4
  Signal Specification1 : SignalSpecification  Dimensions=4
  Subtract : Sum  Inputs=--+
  Unary Minus1 : UnaryMinus
  Unary Minus2 : UnaryMinus
  Vector Concatenate1 : Concatenate  NumInputs=3  Mode=Multidimensional array  ConcatenateDimension=2
  Vector Concatenate2 : Concatenate  NumInputs=4
  Vector Concatenate3 : Concatenate  NumInputs=3  Mode=Multidimensional array
  Vector Concatenate4 : Concatenate  NumInputs=4
  Vector Concatenate5 : Concatenate  Mode=Multidimensional array  ConcatenateDimension=2
  Vector Concatenate6 : Concatenate  Mode=Multidimensional array  ConcatenateDimension=2
  Vector Concatenate8 : Concatenate  NumInputs=3  Mode=Multidimensional array  ConcatenateDimension=2
  Wheel to Body Transform : Subsystem
  Wheel : Outport  VectorParamsAs1DForOutWhenUnconnected=off
  Wheels2Susp : Outport  Port=2  VectorParamsAs1DForOutWhenUnconnected=off
  Omega : Outport  Port=3  VectorParamsAs1DForOutWhenUnconnected=off
  FrntAxlF : Outport  Port=4  VectorParamsAs1DForOutWhenUnconnected=off
  RearAxlF : Outport  Port=5  VectorParamsAs1DForOutWhenUnconnected=off
  <Mz> : Outport  Port=6  VectorParamsAs1DForOutWhenUnconnected=off
  SuspWhlPz : Outport  Port=7  VectorParamsAs1DForOutWhenUnconnected=off
  SuspWhlVz : Outport  Port=8  VectorParamsAs1DForOutWhenUnconnected=off
  wires:
  Fz/1 -> Vector Concatenate8/3
  Vector Concatenate6/1 -> RearAxlF/1
  Vector Concatenate8/1 -> Math Function/1
  Demux/2 -> Vector Concatenate6/1
  Demux1/2 -> Vector Concatenate6/2
  Demux/1 -> Vector Concatenate5/1
  Math Function/1 -> Wheel to Body Transform/1(Forces)
  Bus Selector7/2 -> Signal Specification/1  "<Fx>"
  Vector Concatenate5/1 -> FrntAxlF/1
  Reshape6/1 -> Omega/1
  Demux1/1 -> Vector Concatenate5/2
  Vector Concatenate3/1 -> Wheel to Body Transform/5(WheelAngles)
  Bus Selector7/1 -> [omega], Reshape6/1  "<Omega>"
  Wheel to Body Transform/3(Fz) -> [Fz]
  Bus Selector7/3 -> Signal Specification1/1  "<Fy>"
  Bus Selector7/5 -> Vector Concatenate1/2  "<My>"
  Bus Selector7/7 -> Bus Creator4/4, Wheel to Body Transform/4(<Re>)  "<Re>"
  Bus Selector7/9 -> Unary Minus1/1  "<z>"
  Bus Selector7/8 -> Unary Minus2/1  "<zdot>"
  Bus Selector7/10 -> Bus Creator4/7  "<Kappa>"
  [WheelAngles] -> Bus Creator/1  "WhlAng"
  Bus Creator1/1 -> Wheels2Susp/1
  Bus Creator4/1 -> Bus Creator1/1  "SuspFrame"
  [CamberAngles] -> Bus Creator/2  "WhlCmb"
  Bus Creator/1 -> Bus Creator1/2  "Steering"
  Bus Selector7/11 -> Bus Creator4/8  "<Alpha>"
  Wheel to Body Transform/1(Fx) -> [Fx], Demux/1  "Fx"
  Wheel to Body Transform/2(Fy) -> [Fy], Demux1/1  "Fy"
  Signal Specification/1 -> Vector Concatenate8/1
  Signal Specification1/1 -> Vector Concatenate8/2
  Bus Selector7/4 -> Vector Concatenate1/1  "<Mx>"
  Bus Selector7/6 -> Vector Concatenate1/3  "<Mz>"
  Vector Concatenate1/1 -> Math Function1/1
  DCM/1 -> Wheel to Body Transform/3(DCM)
  Math Function1/1 -> Wheel to Body Transform/2(<M>)
  Constant/1 -> Reshape2/1
  Reshape/1 -> Vector Concatenate3/3
  WhlAng/1 -> Reshape/1, [WheelAngles]
  Reshape1/1 -> Vector Concatenate3/1
  Reshape2/1 -> Vector Concatenate3/2
  WhlCmb/1 -> [CamberAngles], Reshape1/1
  Bus Selector3/2 -> Vector Concatenate2/2  "<Z>"
  Wheel to Body Transform/6(Mz) -> Bus Creator4/3, <Mz>/1  "Mz"
  Bus Selector4/3 -> Vector Concatenate4/3  "<z>"
  Bus Selector4/2 -> Vector Concatenate4/2  "<z>"
  Bus Selector4/4 -> Vector Concatenate4/4  "<z>"
  Reshape4/1 -> SuspWhlVz/1
  Bus Selector4/1 -> Vector Concatenate4/1  "<z>"
  [Fy] -> Bus Creator4/11  "Fy"
  Vector Concatenate2/1 -> Subtract/3
  [Fx] -> Bus Creator4/10  "Fx"
  Wheel to Body Transform/4(Mx) -> Bus Creator4/1  "Mx"
  [omega] -> Bus Creator4/9  "Omega"
  Reshape3/1 -> SuspWhlPz/1
  Bus Selector3/4 -> Vector Concatenate2/4  "<Z>"
  Unary Minus2/1 -> Bus Creator4/5, Reshape4/1  "zdot"
  Wheel to Body Transform/5(My) -> Bus Creator4/2  "My"
  [Fz] -> Bus Creator4/12  "Fz"
  Bus Selector3/1 -> Vector Concatenate2/1  "<Z>"
  Bus Selector3/3 -> Vector Concatenate2/3  "<Z>"
  Vector Concatenate4/1 -> Subtract/2
  Unary Minus1/1 -> Reshape3/1, Bus Creator4/6, Subtract/1  "z"
  Subtract/1 -> Bus Creator4/13, Bus Creator5/1  "dz"
  Veh/1 -> Bus Selector3/1, Bus Selector4/1
  Bus Selector/6 -> Bus Creator5/7  "<My>"
  Bus Selector/1 -> Bus Creator5/2  "<Omega>"
  Bus Selector/10 -> Bus Creator5/11  "<zdot>"
  Bus Selector/3 -> Bus Creator5/4  "<Fy>"
  Bus Selector/2 -> Bus Creator5/3  "<Fx>"
  Bus Selector/4 -> Bus Creator5/5  "<Fz>"
  Bus Selector/8 -> Bus Creator5/9  "<Re>"
  Wheels/1 -> Bus Selector/1, Bus Selector7/1  "TireFrame"
  Bus Creator5/1 -> Bus Creator7/1
  Bus Selector/9 -> Bus Creator5/10  "<z>"
  Bus Selector/11 -> Bus Creator5/12  "<Kappa>"
  Bus Selector/12 -> Bus Creator5/13  "<Alpha>"
  Bus Selector/5 -> Bus Creator5/6  "<Mx>"
  Bus Selector/7 -> Bus Creator5/8  "<Mz>"
  [CamberAngles] -> Bus Creator6/2  "WhlCmb"
  [WheelAngles] -> Bus Creator6/1  "WhlAng"
  Bus Creator7/1 -> Wheel/1  "Wheels"
  Bus Creator6/1 -> Bus Creator7/2  "Steering"

== system V2X_Core_SRI_coding_rate_symbol/VehicleDynamic/Triggered Subsystem ==
  In1 : Inport
  Trigger : TriggerPort  VariantControl=(inherit)
  Out1 : Outport
  wires:
  In1/1 -> Out1/1

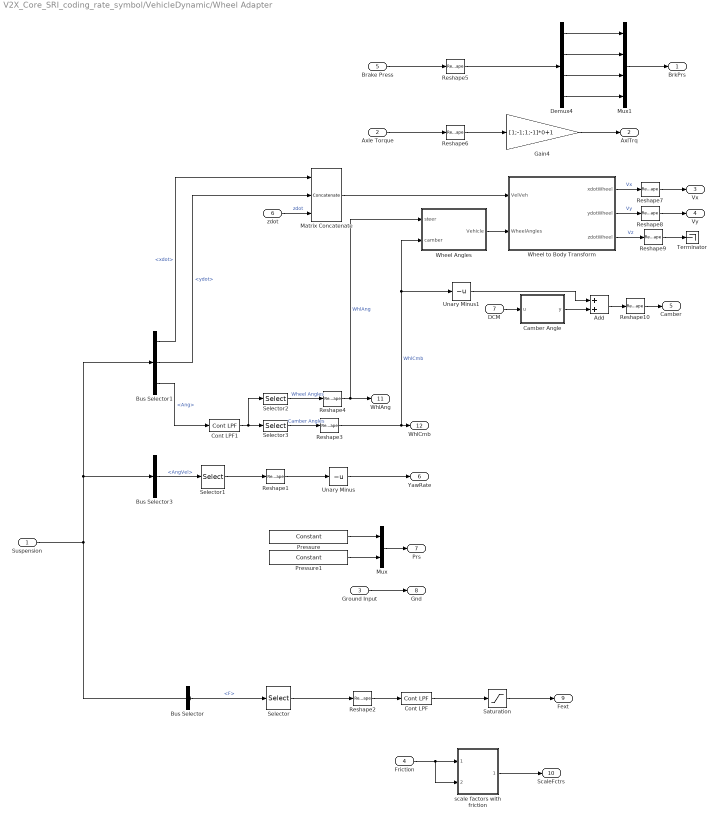
== system V2X_Core_SRI_coding_rate_symbol/VehicleDynamic/Wheel Adapter ==
  Suspension : Inport
  Axle Torque : Inport  Port=2
  Ground Input : Inport  Port=3
  Friction : Inport  Port=4  PortDimensions=4
  Brake Press : Inport  Port=5  Unit=Pa
  zdot : Inport  Port=6
  DCM : Inport  Port=7
  Add : Sum
  Bus Selector : BusSelector  OutputSignals=Whl.F
  Bus Selector1 : BusSelector  OutputSignals=Whl.xdot,Whl.ydot,Whl.Ang
  Bus Selector3 : BusSelector  OutputSignals=Whl.AngVel
  Camber Angle : MATLAB Function  TreatAsAtomicUnit=on
  Cont LPF : autolibutils/Cont LPF  wc=100*2*pi  AbsoluteTolerance=auto  aMode=2
  Cont LPF1 : autolibutils/Cont LPF  wc=100*2*pi  AbsoluteTolerance=1e-2  aMode=2
  Demux4 : Demux
  Gain4 : Gain  Gain=[1;-1;1;-1]*0+1
  Matrix Concatenate : Concatenate  NumInputs=3  Mode=Multidimensional array
  Mux : Mux  Inputs=2
  Mux1 : Mux
  Pressure : vehdynlibtirecommon/Constant  const=Wheels.PressureFront  numWheels=2
  Pressure1 : vehdynlibtirecommon/Constant  const=Wheels.PressureRear  numWheels=2
  Reshape{1..10} (10 alike) : Reshape
  Saturation : Saturate  UpperLimit=inf  LowerLimit=-10*9.81*2000  ZeroCross=off
  Selector : Selector  NumberOfDimensions=2  InputPortWidth=3  IndexOptions=Index vector (dialog),Select all  Indices=[3],1  OutputSizes=1,1
  Selector1 : Selector  NumberOfDimensions=2  InputPortWidth=1  IndexOptions=Index vector (dialog),Select all  Indices=[3],1  OutputSizes=1,1
  Selector2 : Selector  NumberOfDimensions=2  InputPortWidth=3  IndexOptions=Index vector (dialog),Select all  Indices=3,1  OutputSizes=1,1
  Selector3 : Selector  NumberOfDimensions=2  InputPortWidth=3  IndexOptions=Index vector (dialog),Select all  Indices=1,1  OutputSizes=1,1
  Terminator : Terminator
  Unary Minus : UnaryMinus
  Unary Minus1 : UnaryMinus
  Wheel Angles : Subsystem
  Wheel to Body Transform : Subsystem
  scale factors with friction : Subsystem  mask{numWheels=4}
      mask prompts: numWheels "Number of wheels"
  BrkPrs : Outport
  AxlTrq : Outport  Port=2
  Vx : Outport  Port=3
  Vy : Outport  Port=4
  Camber : Outport  Port=5
  YawRate : Outport  Port=6
  Prs : Outport  Port=7
  Gnd : Outport  Port=8
  Fext : Outport  Port=9
  ScaleFctrs : Outport  Port=10
  WhlAng : Outport  Port=11
  WhlCmb : Outport  Port=12
  wires:
  scale factors with friction/1(lambdas) -> ScaleFctrs/1
  Axle Torque/1 -> Reshape6/1
  Brake Press/1 -> Reshape5/1
  Ground Input/1 -> Gnd/1
  Friction/1 -> scale factors with friction/2(lamda_mu_y), scale factors with friction/1(lamda_mu_x)
  Suspension/1 -> Bus Selector/1, Bus Selector3/1, Bus Selector1/1
  Bus Selector1/3 -> Cont LPF1/1  "<Ang>"
  Reshape4/1 -> WhlAng/1, Wheel Angles/1(steer)  "WhlAng"
  Bus Selector1/1 -> Matrix Concatenate/1  "<xdot>"
  Unary Minus/1 -> YawRate/1
  Bus Selector1/2 -> Matrix Concatenate/2  "<ydot>"
  zdot/1 -> Matrix Concatenate/3  "zdot"
  Bus Selector3/1 -> Selector1/1  "<AngVel>"
  Bus Selector/1 -> Selector/1  "<F>"
  Reshape5/1 -> Demux4/1
  Reshape6/1 -> Gain4/1
  Cont LPF1/1 -> Selector3/1, Selector2/1
  Matrix Concatenate/1 -> Wheel to Body Transform/1(VelVeh)
  Selector2/1 -> Reshape4/1  "Wheel Angles"
  Selector1/1 -> Reshape1/1
  Selector/1 -> Reshape2/1
  Add/1 -> Reshape10/1
  Demux4/1 -> Mux1/1
  Reshape9/1 -> Terminator/1
  Demux4/2 -> Mux1/2
  Demux4/3 -> Mux1/3
  Reshape8/1 -> Vy/1
  Demux4/4 -> Mux1/4
  Gain4/1 -> AxlTrq/1
  Selector3/1 -> Reshape3/1  "Camber Angles"
  Reshape1/1 -> Unary Minus/1
  Reshape2/1 -> Cont LPF/1
  Mux1/1 -> BrkPrs/1
  Saturation/1 -> Fext/1
  DCM/1 -> Camber Angle/1(u)
  Reshape3/1 -> WhlCmb/1, Unary Minus1/1, Wheel Angles/2(camber)  "WhlCmb"
  Cont LPF/1 -> Saturation/1
  Reshape10/1 -> Camber/1
  Unary Minus1/1 -> Add/1
  Camber Angle/1(y) -> Add/2
  Wheel to Body Transform/3(zdotWheel) -> Reshape9/1  "Vz"
  Wheel Angles/1(Vehicle) -> Wheel to Body Transform/2(WheelAngles)
  Wheel to Body Transform/1(xdotWheel) -> Reshape7/1  "Vx"
  Wheel to Body Transform/2(ydotWheel) -> Reshape8/1  "Vy"
  Reshape7/1 -> Vx/1
  Pressure/1 -> Mux/1
  Pressure1/1 -> Mux/2
  Mux/1 -> Prs/1

== system V2X_Core_SRI_coding_rate_symbol/DSRC/Queue/Switch Case Action Subsystem ==
  Actor1 : Inport
  Action Port : ActionPort  ActionPortLabel=case [ 0 ]:
  Actor : Outport
  wires:
  Actor1/1 -> Actor/1

== system V2X_Core_SRI_coding_rate_symbol/DSRC/Queue/Switch Case Action Subsystem1 ==
  Actor1 : Inport
  Action Port : ActionPort  ActionPortLabel=case [ 1 ]:
  Out1 : Outport
  wires:
  Actor1/1 -> Out1/1

== system V2X_Core_SRI_coding_rate_symbol/DSRC/Queue/Switch Case Action Subsystem2 ==
  In1 : Inport
  Action Port : ActionPort  ActionPortLabel=case [ 2 ]:
  Out1 : Outport
  wires:
  In1/1 -> Out1/1

== system V2X_Core_SRI_coding_rate_symbol/DSRC/Queue/Switch Case Action Subsystem3 ==
  In1 : Inport
  Action Port : ActionPort  ActionPortLabel=case [ 3 ]:
  Out1 : Outport
  wires:
  In1/1 -> Out1/1

== system V2X_Core_SRI_coding_rate_symbol/DSRC/Queue/Switch Case Action Subsystem4 ==
  In1 : Inport
  Action Port : ActionPort  ActionPortLabel=case [ 4 ]:
  Out1 : Outport
  wires:
  In1/1 -> Out1/1

== system V2X_Core_SRI_coding_rate_symbol/DSRC/Queue/Switch Case Action Subsystem5 ==
  In1 : Inport
  Action Port : ActionPort  ActionPortLabel=case [ 5 ]:
  Out1 : Outport
  wires:
  In1/1 -> Out1/1

== system V2X_Core_SRI_coding_rate_symbol/DSRC/Subsystem/1//2 QPSK ==
  Bits : Inport
  Pilot : Inport  Port=2
  Constant : Constant  Commented=on  Value=zeros(0,1)
  Convolutional Encoder1 : commcnvcod2/Convolutional Encoder  trellis=poly2trellis(7, [171 133])  opMode=Truncated (reset every frame)  DelayedResetAction=on  hasIniStPort=off  hasFinStPort=off  usePuncVector=off  punctureVector=[1; 1; 0; 1; 1; 0]  reset=Unused parameter value
      settings: LibrarySourceBlock=|
      | commhdlcnvcod/Convolutional
      | Encoder
  Gain : Gain  Gain=1/sqrt(5)
  OFDM Modulator : commofdm/OFDM Modulator  StatePerturbationForJacobian=1.0e-05  FFTLength=64  NumGuardBandCarriers=[6; 5]  InsertDCNull=on  PilotInputPort=on  PilotCarrierIndices=[12; 26; 40; 54]  CyclicPrefixLength=16  Windowing=off  WindowLength=1  OversamplingFactor=1  NumSymbols=6  NumTransmitAntennas=1  SimulateUsing=Interpreted execution
  QPSK Modulator Baseband : commdigbbndpm3/QPSK Modulator Baseband  InType=Bit  Enc=Gray  Ph=pi/4  outDtype=double  outWordLen=16  outUDDataType=sfix(16)  outFracLenMode=Best precision  outFracLen=15  outDataTypeStr=double  outLastDataTypeStr=double
      settings: LibrarySourceBlock=|
      | commhdldigbbndpm/QPSK
      | Modulator
      | Baseband
  Random Interleaver : commblkintrlv2/Random Interleaver  StatePerturbationForJacobian=1.0e-05  N=576  seed=12345
  Reshape : Reshape  OutputDimensionality=Customize  OutputDimensions=[48,6]
  Vector Concatenate : Concatenate  Commented=on
  Modulated : Outport
  wires:
  Convolutional Encoder1/1 -> Random Interleaver/1
  Constant/1 -> ?
  Bits/1 -> Convolutional Encoder1/1
  Pilot/1 -> OFDM Modulator/2
  OFDM Modulator/1 -> Modulated/1  "OFDM modulated"
  Random Interleaver/1 -> QPSK Modulator Baseband/1
  Reshape/1 -> OFDM Modulator/1
  QPSK Modulator Baseband/1 -> Gain/1
  Gain/1 -> Reshape/1

== system V2X_Core_SRI_coding_rate_symbol/DSRC/Subsystem/1//2 QPSK1 ==
  Bits : Inport
  Pilot : Inport  Port=2
  Constant : Constant  Commented=on  Value=zeros(96,1)
  Convolutional Encoder1 : commcnvcod2/Convolutional Encoder  trellis=poly2trellis(7, [171 133])  opMode=Truncated (reset every frame)  DelayedResetAction=on  hasIniStPort=off  hasFinStPort=off  usePuncVector=off  punctureVector=[1; 1; 0; 1; 1; 0]  reset=Unused parameter value
      settings: LibrarySourceBlock=|
      | commhdlcnvcod/Convolutional
      | Encoder
  OFDM Modulator : commofdm/OFDM Modulator  StatePerturbationForJacobian=1.0e-05  FFTLength=64  NumGuardBandCarriers=[6; 5]  InsertDCNull=on  PilotInputPort=on  PilotCarrierIndices=[12; 26; 40; 54]  CyclicPrefixLength=16  Windowing=off  WindowLength=1  OversamplingFactor=1  NumSymbols=6  NumTransmitAntennas=1  SimulateUsing=Interpreted execution
  QPSK Modulator Baseband : commdigbbndpm3/QPSK Modulator Baseband  InType=Bit  Enc=Gray  Ph=pi/4  outDtype=double  outWordLen=16  outUDDataType=sfix(16)  outFracLenMode=Best precision  outFracLen=15  outDataTypeStr=double  outLastDataTypeStr=double
      settings: LibrarySourceBlock=|
      | commhdldigbbndpm/QPSK
      | Modulator
      | Baseband
  Random Interleaver : commblkintrlv2/Random Interleaver  StatePerturbationForJacobian=1.0e-05  N=576  seed=12345
  Reshape : Reshape  OutputDimensionality=Customize  OutputDimensions=[48,6]
  Vector Concatenate : Concatenate
  Modulated : Outport
  wires:
  OFDM Modulator/1 -> Modulated/1  "OFDM modulated"
  Pilot/1 -> OFDM Modulator/2
  QPSK Modulator Baseband/1 -> Reshape/1
  Bits/1 -> Convolutional Encoder1/1
  Constant/1 -> Vector Concatenate/2
  Convolutional Encoder1/1 -> Random Interleaver/1
  Reshape/1 -> OFDM Modulator/1
  Random Interleaver/1 -> QPSK Modulator Baseband/1
